simulink model "VehicleThermalSystemSizing"  (R2023b)
settings: Solver=daessc  StartTime=0  StopTime=600  FixedStep=0.2  MaxStep=1  RelTol=1e-3  AbsTol=1e-3
undefined symbols (not defined in the file): air_density, bulb, cabin_H, cabin_L, cabin_W, coolant_pipe_D, coolant_T_init, coolant_tank_volume, CoolingPower_kW, door_or_window_area, duct_W, evap_superheat_temp, inlet, pump_speed_max, refrigerant_massflowrate, RPM_Compressor_nominal, RPM_CondFan, RPM_EvapFan, T_cabin_init, T_set, tube_D, VolFlowrate_CondenserFan, VolFlowRate_CoolantRadiatorFan, VolFlowRate_EvapFan
libraries: fl_lib x128, nesl_utility x45, SimscapeFluids_lib x16, simulink_extras x9
(part 4 of 4)

== system VehicleThermalSystemSizing/Condenser and Fan/Fan/Fan/Fan Drive ==
  Fan On/Off : Inport
  Gain : Gain  Gain=RPM_CondFan
  Ideal Angular Velocity Source : fl_lib/Mechanical/Mechanical Sources/Ideal Angular Velocity Source
  Mechanical Rotational Reference : fl_lib/Mechanical/Rotational Elements/Mechanical Rotational Reference
  Mechanical Power [kW] : Subsystem
      settings: PortSchema="{\"entries\":[{\"content\":{\"sides\":[{\"content\":{\"connectorIds\":[\"LConn1\"]},\"type\":\"ConnectorPlacement.EquallySpacedRectSide\",\"uuid\":\"b1060c97-67a5-45b5-8fe0-0144ebafaeff\"},{\"content\":{\"connectorIds\":[\"RConn1\",\"Out1\"],\"side\":\"RIGHT\"},\"type\":\"ConnectorPlacement.EquallySpacedRectSide\",\"uuid\":\"ebd15156-b3e0-4ce2-8bbb-160ba7fee2c1\"},{\"content\":{\"side\":\"TOP\"},\"type\":\"ConnectorPlacement.EquallySpacedRectSide\",\"uuid\":\"c2873c75-a9ad-4be2-8dbd-a113f7285caf\"}]},\"type\":\"ConnectorPlacement.EquallySpacedConnector\",\"uuid\":\"1871fd39-2348-4d05-b62d-98d5b9ada3fc\"}],\"packageUris\":[\"http://schema.mathworks.com/mf0/Connector/R2020b\"],\"version\":\"1.0\"}"
  Simulink-PS Converter : nesl_utility/Simulink-PS Converter  PhysicalDomain=network_engine_domain  SubClassName=ps_input  LeftPortType=input  RightPortType=output  PseudoPeriodic=off  Frequencies=[]  NoiseDistribution=none  NoiseParameters=[]  Unit=rpm  AffineConversion=off  FilteringAndDerivatives=provide  SimscapeFilterOrder=1  InputFilterTimeConstant=0.001  UdotUserProvided=0
  Transfer Fcn (with initial outputs) : simulink_extras/Additional Linear/Transfer Fcn (with initial outputs)  N=[1]  D="[2  1]"  Y0=0  U0=0
      settings: AttributesFormatString=|
      | Initial U= %<U0>
      | Initial Y=%<Y0>
  R : PMIOPort  Side=Left
  C : PMIOPort  Port=2  Side=Right
  Mech Power [kW] : Outport
  wires:
  Fan On/Off/1 -> Transfer Fcn (with initial outputs)/1
  Mechanical Power [kW]/1(Power [kW]) -> Mech Power [kW]/1
  Gain/1 -> Simulink-PS Converter/1
  Transfer Fcn (with initial outputs)/1 -> Gain/1
  connections:
  Ideal Angular Velocity Source/RConn1 -- Simulink-PS Converter/RConn1
  C/RConn1 -- Mechanical Rotational Reference/LConn1 -- Ideal Angular Velocity Source/RConn2
  R/RConn1 -- Mechanical Power [kW]/LConn1
  Mechanical Power [kW]/RConn1 -- Ideal Angular Velocity Source/LConn1

== system VehicleThermalSystemSizing/Condenser and Fan/Fan/Fan (Simple)/Power calculation ==
  note: Fan power calculation
  Enthalpy change [J/kg] : fl_lib/Physical Signals/Functions/PS Subtract
  Enthalpy in : fl_lib/Moist Air/Sensors/Thermodynamic Properties Sensor (MA)  measurement_mass_spec=foundation.enum.measurement_mass_spec.mixture  enthalpy=true  enthalpy_reference=foundation.enum.EnthalpyReference.PropertyTables  density=false  specific_heat=false  entropy=false
      settings: InternalSimscapePortConfiguration="{\"Bottom\":[],\"Left\":[{\"id\":\"A\",\"label\":\"A\",\"type\":\"foundation.moist_air.moist_air\"}],\"Right\":[{\"id\":\"H\",\"label\":\"h\",\"type\":\"output\"}],\"Top\":[]}"
  "Enthalpy out " : fl_lib/Moist Air/Sensors/Thermodynamic Properties Sensor (MA)  measurement_mass_spec=foundation.enum.measurement_mass_spec.mixture  enthalpy=true  enthalpy_reference=foundation.enum.EnthalpyReference.PropertyTables  density=false  specific_heat=false  entropy=false
      settings: InternalSimscapePortConfiguration="{\"Bottom\":[],\"Left\":[{\"id\":\"A\",\"label\":\"A\",\"type\":\"foundation.moist_air.moist_air\"}],\"Right\":[{\"id\":\"H\",\"label\":\"h\",\"type\":\"output\"}],\"Top\":[]}"
  Fan power : fl_lib/Physical Signals/Functions/PS Product
  "MassFlowRate [kg/s] " : fl_lib/Moist Air/Sensors/Flow Rate Sensor (MA)  mass_flow_measure=true  volumetric_flow_measure=false  volumetric_flow_conditions=foundation.enum.volumetric_flow_conditions.actual  p_std=0.101325 MPa  T_std=20 degC  RH_std=0.65  energy_flow_measure=false  vapor_flow_measure=false  gas_flow_measure=false
      settings: InternalSimscapePortConfiguration="{\"Bottom\":[],\"Left\":[{\"id\":\"A\",\"label\":\"A\",\"type\":\"foundation.moist_air.moist_air\"}],\"Right\":[{\"id\":\"B\",\"label\":\"B\",\"type\":\"foundation.moist_air.moist_air\"},{\"id\":\"M\",\"label\":\"M\",\"type\":\"output\"}],\"Top\":[]}"
  PS-Simulink Converter : nesl_utility/PS-Simulink Converter  PhysicalDomain=network_engine_domain  SubClassName=ps_output  LeftPortType=input  RightPortType=output  PseudoPeriodic=off  Frequencies=[]  VectorFormat=1-D array  Unit=kW  AffineConversion=off
  B : PMIOPort  Side=Left
  Outflow : PMIOPort  Port=2  Side=Left
  A : PMIOPort  Port=3  Side=Right
  Power : Outport
  wires:
  PS-Simulink Converter/1 -> Power/1
  connections:
  Fan power/RConn1 -- PS-Simulink Converter/LConn1
  Enthalpy in/RConn1 -- Enthalpy change [J/kg]/LConn2
  A/RConn1 -- "MassFlowRate [kg/s] "/LConn1 -- Enthalpy in/LConn1
  Enthalpy change [J/kg]/RConn1 -- Fan power/LConn2
  Outflow/RConn1 -- "Enthalpy out "/LConn1
  "Enthalpy out "/RConn1 -- Enthalpy change [J/kg]/LConn1
  "MassFlowRate [kg/s] "/RConn1 -- B/RConn1
  "MassFlowRate [kg/s] "/RConn2 -- Fan power/LConn1

== system VehicleThermalSystemSizing/Coolant Circuit/Fan and Radiator/Direct connect/Power calculation ==
  note: Fan power calculation
  Enthalpy change [J/kg] : fl_lib/Physical Signals/Functions/PS Subtract
  Enthalpy in : fl_lib/Moist Air/Sensors/Thermodynamic Properties Sensor (MA)  measurement_mass_spec=foundation.enum.measurement_mass_spec.mixture  enthalpy=true  enthalpy_reference=foundation.enum.EnthalpyReference.PropertyTables  density=false  specific_heat=false  entropy=false
      settings: InternalSimscapePortConfiguration="{\"Bottom\":[],\"Left\":[{\"id\":\"A\",\"label\":\"A\",\"type\":\"foundation.moist_air.moist_air\"}],\"Right\":[{\"id\":\"H\",\"label\":\"h\",\"type\":\"output\"}],\"Top\":[]}"
  "Enthalpy out " : fl_lib/Moist Air/Sensors/Thermodynamic Properties Sensor (MA)  measurement_mass_spec=foundation.enum.measurement_mass_spec.mixture  enthalpy=true  enthalpy_reference=foundation.enum.EnthalpyReference.PropertyTables  density=false  specific_heat=false  entropy=false
      settings: InternalSimscapePortConfiguration="{\"Bottom\":[],\"Left\":[{\"id\":\"A\",\"label\":\"A\",\"type\":\"foundation.moist_air.moist_air\"}],\"Right\":[{\"id\":\"H\",\"label\":\"h\",\"type\":\"output\"}],\"Top\":[]}"
  Fan power : fl_lib/Physical Signals/Functions/PS Product
  "MassFlowRate [kg/s] " : fl_lib/Moist Air/Sensors/Flow Rate Sensor (MA)  mass_flow_measure=true  volumetric_flow_measure=false  volumetric_flow_conditions=foundation.enum.volumetric_flow_conditions.actual  p_std=0.101325 MPa  T_std=20 degC  RH_std=0.65  energy_flow_measure=false  vapor_flow_measure=false  gas_flow_measure=false
      settings: InternalSimscapePortConfiguration="{\"Bottom\":[],\"Left\":[{\"id\":\"A\",\"label\":\"A\",\"type\":\"foundation.moist_air.moist_air\"}],\"Right\":[{\"id\":\"B\",\"label\":\"B\",\"type\":\"foundation.moist_air.moist_air\"},{\"id\":\"M\",\"label\":\"M\",\"type\":\"output\"}],\"Top\":[]}"
  PS-Simulink Converter : nesl_utility/PS-Simulink Converter  PhysicalDomain=network_engine_domain  SubClassName=ps_output  LeftPortType=input  RightPortType=output  PseudoPeriodic=off  Frequencies=[]  VectorFormat=1-D array  Unit=kW  AffineConversion=off
  B : PMIOPort  Side=Left
  A : PMIOPort  Port=2  Side=Right
  Outflow : PMIOPort  Port=3  Side=Right
  Power : Outport
  wires:
  PS-Simulink Converter/1 -> Power/1
  connections:
  "MassFlowRate [kg/s] "/RConn2 -- Fan power/LConn1
  "Enthalpy out "/RConn1 -- Enthalpy change [J/kg]/LConn1
  Outflow/RConn1 -- "Enthalpy out "/LConn1
  Enthalpy change [J/kg]/RConn1 -- Fan power/LConn2
  A/RConn1 -- "MassFlowRate [kg/s] "/LConn1 -- Enthalpy in/LConn1
  Enthalpy in/RConn1 -- Enthalpy change [J/kg]/LConn2
  Fan power/RConn1 -- PS-Simulink Converter/LConn1
  "MassFlowRate [kg/s] "/RConn1 -- B/RConn1

== system VehicleThermalSystemSizing/Coolant Circuit/Fan and Radiator/Fan and Radiator/Power calculation ==
  note: Fan power calculation
  Enthalpy change [J/kg] : fl_lib/Physical Signals/Functions/PS Subtract
  Enthalpy in : fl_lib/Moist Air/Sensors/Thermodynamic Properties Sensor (MA)  measurement_mass_spec=foundation.enum.measurement_mass_spec.mixture  enthalpy=true  enthalpy_reference=foundation.enum.EnthalpyReference.PropertyTables  density=false  specific_heat=false  entropy=false
      settings: InternalSimscapePortConfiguration="{\"Bottom\":[],\"Left\":[{\"id\":\"A\",\"label\":\"A\",\"type\":\"foundation.moist_air.moist_air\"}],\"Right\":[{\"id\":\"H\",\"label\":\"h\",\"type\":\"output\"}],\"Top\":[]}"
  "Enthalpy out " : fl_lib/Moist Air/Sensors/Thermodynamic Properties Sensor (MA)  measurement_mass_spec=foundation.enum.measurement_mass_spec.mixture  enthalpy=true  enthalpy_reference=foundation.enum.EnthalpyReference.PropertyTables  density=false  specific_heat=false  entropy=false
      settings: InternalSimscapePortConfiguration="{\"Bottom\":[],\"Left\":[{\"id\":\"A\",\"label\":\"A\",\"type\":\"foundation.moist_air.moist_air\"}],\"Right\":[{\"id\":\"H\",\"label\":\"h\",\"type\":\"output\"}],\"Top\":[]}"
  Fan power : fl_lib/Physical Signals/Functions/PS Product
  "MassFlowRate [kg/s] " : fl_lib/Moist Air/Sensors/Flow Rate Sensor (MA)  mass_flow_measure=true  volumetric_flow_measure=false  volumetric_flow_conditions=foundation.enum.volumetric_flow_conditions.actual  p_std=0.101325 MPa  T_std=20 degC  RH_std=0.65  energy_flow_measure=false  vapor_flow_measure=false  gas_flow_measure=false
      settings: InternalSimscapePortConfiguration="{\"Bottom\":[],\"Left\":[{\"id\":\"A\",\"label\":\"A\",\"type\":\"foundation.moist_air.moist_air\"}],\"Right\":[{\"id\":\"B\",\"label\":\"B\",\"type\":\"foundation.moist_air.moist_air\"},{\"id\":\"M\",\"label\":\"M\",\"type\":\"output\"}],\"Top\":[]}"
  PS-Simulink Converter : nesl_utility/PS-Simulink Converter  PhysicalDomain=network_engine_domain  SubClassName=ps_output  LeftPortType=input  RightPortType=output  PseudoPeriodic=off  Frequencies=[]  VectorFormat=1-D array  Unit=kW  AffineConversion=off
  B : PMIOPort  Side=Left
  A : PMIOPort  Port=2  Side=Right
  Outflow : PMIOPort  Port=3  Side=Right
  Power : Outport
  wires:
  PS-Simulink Converter/1 -> Power/1
  connections:
  "MassFlowRate [kg/s] "/RConn2 -- Fan power/LConn1
  "Enthalpy out "/RConn1 -- Enthalpy change [J/kg]/LConn1
  Outflow/RConn1 -- "Enthalpy out "/LConn1
  Enthalpy change [J/kg]/RConn1 -- Fan power/LConn2
  A/RConn1 -- "MassFlowRate [kg/s] "/LConn1 -- Enthalpy in/LConn1
  Enthalpy in/RConn1 -- Enthalpy change [J/kg]/LConn2
  Fan power/RConn1 -- PS-Simulink Converter/LConn1
  "MassFlowRate [kg/s] "/RConn1 -- B/RConn1

== system VehicleThermalSystemSizing/Evaporator and Blower Fan/Fan/Fan/Fan Drive ==
  Blower Fan On/Off : Inport
  Gain : Gain  Gain=RPM_EvapFan
  Ideal Angular Velocity Source : fl_lib/Mechanical/Mechanical Sources/Ideal Angular Velocity Source
  Mechanical Rotational Reference : fl_lib/Mechanical/Rotational Elements/Mechanical Rotational Reference
  Mechanical Power [kW] : Subsystem
      settings: PortSchema="{\"entries\":[{\"content\":{\"sides\":[{\"content\":{\"connectorIds\":[\"LConn1\"]},\"type\":\"ConnectorPlacement.EquallySpacedRectSide\",\"uuid\":\"b1060c97-67a5-45b5-8fe0-0144ebafaeff\"},{\"content\":{\"connectorIds\":[\"RConn1\",\"Out1\"],\"side\":\"RIGHT\"},\"type\":\"ConnectorPlacement.EquallySpacedRectSide\",\"uuid\":\"ebd15156-b3e0-4ce2-8bbb-160ba7fee2c1\"},{\"content\":{\"side\":\"TOP\"},\"type\":\"ConnectorPlacement.EquallySpacedRectSide\",\"uuid\":\"c2873c75-a9ad-4be2-8dbd-a113f7285caf\"}]},\"type\":\"ConnectorPlacement.EquallySpacedConnector\",\"uuid\":\"1871fd39-2348-4d05-b62d-98d5b9ada3fc\"}],\"packageUris\":[\"http://schema.mathworks.com/mf0/Connector/R2020b\"],\"version\":\"1.0\"}"
  Simulink-PS Converter : nesl_utility/Simulink-PS Converter  PhysicalDomain=network_engine_domain  SubClassName=ps_input  LeftPortType=input  RightPortType=output  PseudoPeriodic=off  Frequencies=[]  NoiseDistribution=none  NoiseParameters=[]  Unit=rpm  AffineConversion=off  FilteringAndDerivatives=provide  SimscapeFilterOrder=1  InputFilterTimeConstant=0.001  UdotUserProvided=0
  Transfer Fcn (with initial outputs) : simulink_extras/Additional Linear/Transfer Fcn (with initial outputs)  N=[1]  D="[2  1]"  Y0=0  U0=0
      settings: AttributesFormatString=|
      | Initial U= %<U0>
      | Initial Y=%<Y0>
  C : PMIOPort  Side=Left
  R : PMIOPort  Port=2  Side=Right
  Power [kW] : Outport
  wires:
  Blower Fan On/Off/1 -> Transfer Fcn (with initial outputs)/1
  Mechanical Power [kW]/1(Power [kW]) -> Power [kW]/1
  Gain/1 -> Simulink-PS Converter/1
  Transfer Fcn (with initial outputs)/1 -> Gain/1
  connections:
  Ideal Angular Velocity Source/RConn1 -- Simulink-PS Converter/RConn1
  Ideal Angular Velocity Source/RConn2 -- Mechanical Rotational Reference/LConn1 -- C/RConn1
  Mechanical Power [kW]/LConn1 -- Ideal Angular Velocity Source/LConn1
  R/RConn1 -- Mechanical Power [kW]/RConn1

== system VehicleThermalSystemSizing/Evaporator and Blower Fan/Fan/Fan (Simple)/Power calculation ==
  note: Fan power calculation
  Enthalpy change [J/kg] : fl_lib/Physical Signals/Functions/PS Subtract
  Enthalpy in : fl_lib/Moist Air/Sensors/Thermodynamic Properties Sensor (MA)  measurement_mass_spec=foundation.enum.measurement_mass_spec.mixture  enthalpy=true  enthalpy_reference=foundation.enum.EnthalpyReference.PropertyTables  density=true  specific_heat=true  entropy=true
      settings: InternalSimscapePortConfiguration="{\"Bottom\":[{\"id\":\"CP\",\"label\":\"cp\",\"type\":\"output\"},{\"id\":\"S\",\"label\":\"s\",\"type\":\"output\"}],\"Left\":[{\"id\":\"A\",\"label\":\"A\",\"type\":\"foundation.moist_air.moist_air\"}],\"Right\":[{\"id\":\"H\",\"label\":\"h\",\"type\":\"output\"},{\"id\":\"RHO\",\"label\":\"ρ\",\"type\":\"output\"}],\"Top\":[]}"
  "Enthalpy out " : fl_lib/Moist Air/Sensors/Thermodynamic Properties Sensor (MA)  measurement_mass_spec=foundation.enum.measurement_mass_spec.mixture  enthalpy=true  enthalpy_reference=foundation.enum.EnthalpyReference.PropertyTables  density=true  specific_heat=true  entropy=true
      settings: InternalSimscapePortConfiguration="{\"Bottom\":[{\"id\":\"CP\",\"label\":\"cp\",\"type\":\"output\"},{\"id\":\"S\",\"label\":\"s\",\"type\":\"output\"}],\"Left\":[{\"id\":\"A\",\"label\":\"A\",\"type\":\"foundation.moist_air.moist_air\"}],\"Right\":[{\"id\":\"H\",\"label\":\"h\",\"type\":\"output\"},{\"id\":\"RHO\",\"label\":\"ρ\",\"type\":\"output\"}],\"Top\":[]}"
  Fan power : fl_lib/Physical Signals/Functions/PS Product
  "MassFlowRate [kg/s] " : fl_lib/Moist Air/Sensors/Flow Rate Sensor (MA)  mass_flow_measure=true  volumetric_flow_measure=false  volumetric_flow_conditions=foundation.enum.volumetric_flow_conditions.actual  p_std=0.101325 MPa  T_std=20 degC  RH_std=0.65  energy_flow_measure=false  vapor_flow_measure=false  gas_flow_measure=false
      settings: InternalSimscapePortConfiguration="{\"Bottom\":[],\"Left\":[{\"id\":\"A\",\"label\":\"A\",\"type\":\"foundation.moist_air.moist_air\"}],\"Right\":[{\"id\":\"B\",\"label\":\"B\",\"type\":\"foundation.moist_air.moist_air\"},{\"id\":\"M\",\"label\":\"M\",\"type\":\"output\"}],\"Top\":[]}"
  PS-Simulink Converter : nesl_utility/PS-Simulink Converter  PhysicalDomain=network_engine_domain  SubClassName=ps_output  LeftPortType=input  RightPortType=output  PseudoPeriodic=off  Frequencies=[]  VectorFormat=1-D array  Unit=kW  AffineConversion=off
  B : PMIOPort  Side=Left
  Outflow : PMIOPort  Port=2  Side=Left
  A : PMIOPort  Port=3  Side=Right
  Power : Outport
  wires:
  PS-Simulink Converter/1 -> Power/1
  connections:
  Fan power/RConn1 -- PS-Simulink Converter/LConn1
  Enthalpy in/RConn1 -- Enthalpy change [J/kg]/LConn2
  Enthalpy in/LConn1 -- A/RConn1 -- "MassFlowRate [kg/s] "/LConn1
  Enthalpy change [J/kg]/RConn1 -- Fan power/LConn2
  Outflow/RConn1 -- "Enthalpy out "/LConn1
  "Enthalpy out "/RConn1 -- Enthalpy change [J/kg]/LConn1
  "MassFlowRate [kg/s] "/RConn1 -- B/RConn1
  "MassFlowRate [kg/s] "/RConn2 -- Fan power/LConn1

== system VehicleThermalSystemSizing/Compressor/Compressor/Compressor (detailed)/Compressor Drive and Control/Compressor drive ==
  note: The saturation block makes sure the fluid flow rate does not go to zero, for numerical stability
  Compressor ON/OFF : Inport
  Saturation : Saturate  UpperLimit=inf  LowerLimit=10
      settings: AttributesFormatString=|
      | UpperLimit= %<UpperLimit>
      | LowerLimit= %<LowerLimit>
  Shaft Speed : Gain  Gain=RPM_Compressor_nominal
  Simulink-PS Converter : nesl_utility/Simulink-PS Converter  PhysicalDomain=network_engine_domain  SubClassName=ps_input  LeftPortType=input  RightPortType=output  PseudoPeriodic=off  Frequencies=[]  NoiseDistribution=none  NoiseParameters=[]  Unit=rpm  AffineConversion=off  FilteringAndDerivatives=provide  SimscapeFilterOrder=1  InputFilterTimeConstant=0.1  UdotUserProvided=0
  Speed Source : fl_lib/Mechanical/Mechanical Sources/Ideal Angular Velocity Source
  Transfer Fcn (with initial outputs) : simulink_extras/Additional Linear/Transfer Fcn (with initial outputs)  N=[1]  D="[2  1]"  Y0=0  U0=0
      settings: AttributesFormatString=|
      | Initial U= %<U0>
      | Initial Y=%<Y0>
  R : PMIOPort  Side=Right
  C : PMIOPort  Port=2  Side=Right
  wires:
  Shaft Speed/1 -> Saturation/1
  Compressor ON/OFF/1 -> Transfer Fcn (with initial outputs)/1
  Transfer Fcn (with initial outputs)/1 -> Shaft Speed/1
  Saturation/1 -> Simulink-PS Converter/1
  connections:
  Simulink-PS Converter/RConn1 -- Speed Source/RConn1
  C/RConn1 -- Speed Source/RConn2
  R/RConn1 -- Speed Source/LConn1

== system VehicleThermalSystemSizing/Compressor/Compressor/Compressor (detailed)/Compressor Drive and Control/Mechanical Power [kW] ==
  Ideal Rotational Motion Sensor : fl_lib/Mechanical/Mechanical Sensors/Ideal Rotational Motion Sensor  reference=foundation.enum.MeasurementReference.difference  acceleration_port=false  velocity_port=true  position_port=true  wrap_angle=false  offset=0 rad
  Mechanical Rotational Reference1 : fl_lib/Mechanical/Rotational Elements/Mechanical Rotational Reference
  PS-Simulink Converter : nesl_utility/PS-Simulink Converter  PhysicalDomain=network_engine_domain  SubClassName=ps_output  LeftPortType=input  RightPortType=output  PseudoPeriodic=off  Frequencies=[]  VectorFormat=inherit  Unit=kW  AffineConversion=off
  Power = T x w : fl_lib/Physical Signals/Functions/PS Product
  Torque Sensor : fl_lib/Mechanical/Mechanical Sensors/Ideal Torque Sensor
  R : PMIOPort  Side=Left
  C : PMIOPort  Port=2  Side=Right
  Power [kW] : Outport
  wires:
  PS-Simulink Converter/1 -> Power [kW]/1
  connections:
  Ideal Rotational Motion Sensor/RConn2 -- Power = T x w/LConn1
  Ideal Rotational Motion Sensor/LConn1 -- Torque Sensor/RConn1 -- C/RConn1
  Ideal Rotational Motion Sensor/RConn1 -- Mechanical Rotational Reference1/LConn1
  PS-Simulink Converter/LConn1 -- Power = T x w/RConn1
  Torque Sensor/LConn1 -- R/RConn1
  Power = T x w/LConn2 -- Torque Sensor/RConn2

== system VehicleThermalSystemSizing/Condenser and Fan/Fan/Fan/Fan Drive/Mechanical Power [kW] ==
  Ideal Rotational Motion Sensor : fl_lib/Mechanical/Mechanical Sensors/Ideal Rotational Motion Sensor  reference=foundation.enum.MeasurementReference.difference  acceleration_port=false  velocity_port=true  position_port=false  wrap_angle=false  offset=0 rad
      settings: InternalSimscapePortConfiguration="{\"Bottom\":[],\"Left\":[{\"id\":\"R\",\"label\":\"R\",\"type\":\"foundation.mechanical.rotational.rotational\"}],\"Right\":[{\"id\":\"C\",\"label\":\"C\",\"type\":\"foundation.mechanical.rotational.rotational\"},{\"id\":\"W\",\"label\":\"W\",\"type\":\"output\"}],\"Top\":[]}"
  Mechanical Rotational Reference1 : fl_lib/Mechanical/Rotational Elements/Mechanical Rotational Reference
  PS-Simulink Converter : nesl_utility/PS-Simulink Converter  PhysicalDomain=network_engine_domain  SubClassName=ps_output  LeftPortType=input  RightPortType=output  PseudoPeriodic=off  Frequencies=[]  VectorFormat=inherit  Unit=kW  AffineConversion=off
  Power = T x w : fl_lib/Physical Signals/Functions/PS Product
  Torque Sensor : fl_lib/Mechanical/Mechanical Sensors/Ideal Torque Sensor
  R : PMIOPort  Side=Left
  C : PMIOPort  Port=2  Side=Right
  Power [kW] : Outport
  wires:
  PS-Simulink Converter/1 -> Power [kW]/1
  connections:
  Ideal Rotational Motion Sensor/RConn2 -- Power = T x w/LConn1
  C/RConn1 -- Torque Sensor/LConn1 -- Ideal Rotational Motion Sensor/LConn1
  Ideal Rotational Motion Sensor/RConn1 -- Mechanical Rotational Reference1/LConn1
  PS-Simulink Converter/LConn1 -- Power = T x w/RConn1
  Torque Sensor/RConn1 -- R/RConn1
  Torque Sensor/RConn2 -- Power = T x w/LConn2

== system VehicleThermalSystemSizing/Evaporator and Blower Fan/Fan/Fan/Fan Drive/Mechanical Power [kW] ==
  Ideal Rotational Motion Sensor : fl_lib/Mechanical/Mechanical Sensors/Ideal Rotational Motion Sensor  reference=foundation.enum.MeasurementReference.difference  acceleration_port=false  velocity_port=true  position_port=true  wrap_angle=false  offset=0 rad
  Mechanical Rotational Reference1 : fl_lib/Mechanical/Rotational Elements/Mechanical Rotational Reference
  PS-Simulink Converter : nesl_utility/PS-Simulink Converter  PhysicalDomain=network_engine_domain  SubClassName=ps_output  LeftPortType=input  RightPortType=output  PseudoPeriodic=off  Frequencies=[]  VectorFormat=inherit  Unit=kW  AffineConversion=off
  Power = T x w : fl_lib/Physical Signals/Functions/PS Product
  Torque Sensor : fl_lib/Mechanical/Mechanical Sensors/Ideal Torque Sensor
  R : PMIOPort  Side=Left
  C : PMIOPort  Port=2  Side=Right
  Power [kW] : Outport
  wires:
  PS-Simulink Converter/1 -> Power [kW]/1
  connections:
  Ideal Rotational Motion Sensor/RConn2 -- Power = T x w/LConn1
  C/RConn1 -- Torque Sensor/RConn1 -- Ideal Rotational Motion Sensor/LConn1
  Ideal Rotational Motion Sensor/RConn1 -- Mechanical Rotational Reference1/LConn1
  PS-Simulink Converter/LConn1 -- Power = T x w/RConn1
  Torque Sensor/LConn1 -- R/RConn1
  Power = T x w/LConn2 -- Torque Sensor/RConn2
